simulink model "nonlinear_system"  (R2024b)
settings: Solver=VariableStepAuto  StartTime=0.0  StopTime=2  RelTol=1e-3
values from neighbouring files (symbols this model uses):
  Cd = [0 1]    [mpc3.m]
  Cr = 87342    [mpc3.m]    (also in prueba_mpc.m; prueba_mpc2.m)
  m = 1400    [mpc3.m]    (also in prueba_mpc.m; prueba_mpc2.m)
  R = 1    [prueba_mpc.m]    (also in prueba_mpc2.m)
undefined symbols (not defined in the file or in its folder): Af, FN, g, mode, mu1, mu2, mu3, omega, theta
settings Model: Creator=inaki  LastModifiedBy=inaki

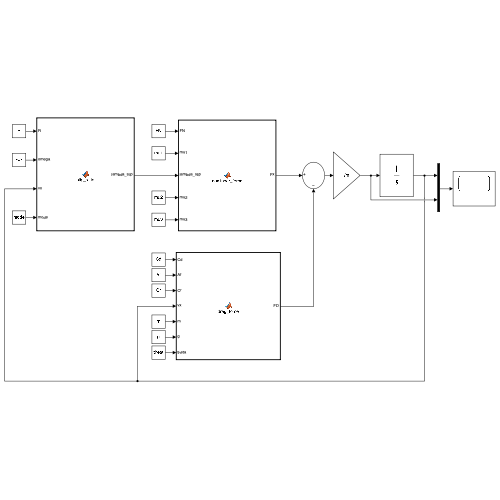
[thumbnail: Simulink's stored preview of the top-level diagram]
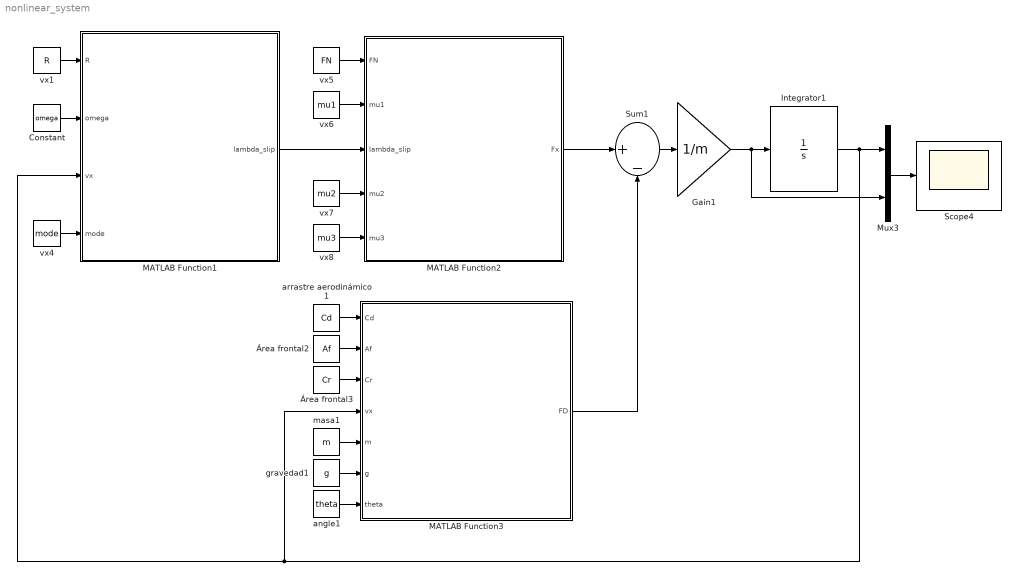
== system nonlinear_system ==
  Constant : Constant  Value=omega
  Gain1 : Gain  Gain=1/m
  Integrator1 : Integrator  ZeroCross=off
  MATLAB Function1 : MATLAB Function  TreatAsAtomicUnit=on
  MATLAB Function2 : MATLAB Function  TreatAsAtomicUnit=on
  MATLAB Function3 : MATLAB Function  TreatAsAtomicUnit=on
  Mux3 : Mux  Inputs=2
  Scope4 : Scope
  Sum1 : Sum  Inputs=|+-
  angle1 : Constant  Value=theta  VectorParams1D=off
  arrastre aerodinámico1 : Constant  Value=Cd  VectorParams1D=off
  gravedad1 : Constant  Value=g  VectorParams1D=off
  masa1 : Constant  Value=m  VectorParams1D=off
  vx1 : Constant  Value=R  VectorParams1D=off  SampleTime=R
  vx4 : Constant  Value=mode  VectorParams1D=off  SampleTime=mode
  vx5 : Constant  Value=FN  VectorParams1D=off  SampleTime=R
  vx6 : Constant  Value=mu1  VectorParams1D=off  SampleTime=R
  vx7 : Constant  Value=mu2  VectorParams1D=off  SampleTime=R
  vx8 : Constant  Value=mu3  VectorParams1D=off  SampleTime=R
  Área frontal2 : Constant  Value=Af  VectorParams1D=off
  Área frontal3 : Constant  Value=Cr  VectorParams1D=off
  wires:
  Área frontal2/1 -> MATLAB Function3/2(Af)
  vx5/1 -> MATLAB Function2/1(FN)
  Gain1/1 -> Integrator1/1, Mux3/2
  vx7/1 -> MATLAB Function2/4(mu2)
  MATLAB Function2/1(Fx) -> Sum1/1
  Mux3/1 -> Scope4/1
  Constant/1 -> MATLAB Function1/2(omega)
  vx8/1 -> MATLAB Function2/5(mu3)
  vx1/1 -> MATLAB Function1/1(R)
  Área frontal3/1 -> MATLAB Function3/3(Cr)
  Integrator1/1 -> MATLAB Function1/3(vx), MATLAB Function3/4(vx), Mux3/1
  vx4/1 -> MATLAB Function1/4(mode)
  vx6/1 -> MATLAB Function2/2(mu1)
  MATLAB Function1/1(lambda_slip) -> MATLAB Function2/3(lambda_slip)
  MATLAB Function3/1(FD) -> Sum1/2
  gravedad1/1 -> MATLAB Function3/6(g)
  Sum1/1 -> Gain1/1
  angle1/1 -> MATLAB Function3/7(theta)
  arrastre aerodinámico1/1 -> MATLAB Function3/1(Cd)
  masa1/1 -> MATLAB Function3/5(m)

== matlab function nonlinear_system/MATLAB Function1 ==
  data: R input; lambda_slip output; omega input; vx input; mode input
function lambda_slip = slip_ratio(R,omega,vx,mode)
    epsilon = 1e-6; % Small threshold for near-zero values

    if abs(vx) < epsilon
        vx = sign(vx) * epsilon;
    end
    if abs(omega) < epsilon
        omega = sign(omega) * epsilon;
    end

    if mode == 1  % 'braking'
        if abs(R * omega - vx) < epsilon || abs(vx) < epsilon
            lambda_slip = 0;
        else
            lambda_slip = (R * omega - vx) / vx;
        end
    elseif mode == 2  % 'acceleration'
        if abs(R * omega - vx) < epsilon || abs(R * omega) < epsilon
            lambda_slip = 0;
        else
            lambda_slip = (R * omega - vx) / (R * omega);
        end
    else
        lambda_slip = 1;  
    end
end

== matlab function nonlinear_system/MATLAB Function2 ==
  data: FN input; mu1 input; lambda_slip input; Fx output; mu2 input; mu3 input
function Fx = nonlinear_force(FN,mu1,lambda_slip,mu2,mu3)
    mu_lambda = sign(lambda_slip) * (mu1 * (1 - exp(-abs(lambda_slip) * mu2)) - abs(lambda_slip) * mu3);
    Fx = mu_lambda * FN;
end

== matlab function nonlinear_system/MATLAB Function3 ==
  data: Cd input; Af input; Cr input; vx input; FD output; m input; g input; theta input
function FD = drag_force(Cd,Af,Cr,vx,m,g,theta)
    rho = 1.225; 
    drag_term = 0.5 * rho * Cd * Af * vx^2;
    if abs(vx) < 1e-3
        drag_term = 0;  
    end


    rolling_resistance = Cr * m * g * cos(theta);

 
    FD = drag_term + rolling_resistance;


    if ~isfinite(FD)
        FD = 0; 
    end
end
